simulink model "regulador_estabilidade"  (Simulink 7.9)
settings: Solver=ode4  SolverMode=SingleTasking  StartTime=0.0  StopTime=12  FixedStep=0.1  RelTol=1e-3
StartFcn:
  | clc
undefined symbols (not defined in the file or in its folder): A, Ac, Aeq, Aqp, B, Bc, Hn, Hqp, Phiu, Q, R, T
settings Model: Creator=Kawakami  LastModifiedBy=Kawakami
settings DataIOCC: SignalLoggingName=sigsOut
settings OptimizationCC: BooleanDataType=off
settings DebuggingCC: SaveWithParameterizedLinksMsg=none  SignalResolutionControl=TryResolveAllWithWarning  SolverPrmCheckMsg=none  MultiTaskDSMMsg=warning  MultiTaskCondExecSysMsg=none  FcnCallInpInsideContextMsg=Use local settings  StrictBusMsg=None
settings HardwareCC: TargetUnknown=on
settings RTWCC: IncludeERTFirstTime=on
settings GRTTargetCC: CombineOutputUpdateFcns=off  GRTInterface=on

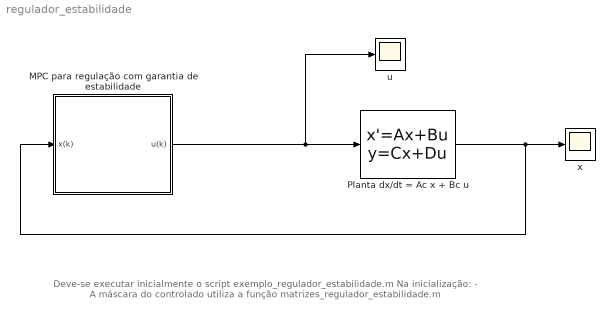
== system regulador_estabilidade ==
  note: Deve-se executar inicialmente o script exemplo_regulador_estabilidade.m
      |
      | Na inicialização:
      | - A máscara do controlado utiliza a função matrizes_regulador_estabilidade.m
  MPC para regulação com garantia de estabilidade : Subsystem  mask{Q=Q, R=R, N=10, A=A, B=B, ulim=[-0.2 0.2], xlim=[-2 2;-2 2], T=T}
      mask prompts: Q "Matriz de pesos dos estados Q (n x n)"; R "Matriz de pesos dos controle (R) (p x p)"; N "Horizonte de Predição (N)"; A "Matriz A (n x n)"; B "Matriz B (n x p)"; ulim "[umin, umax] (p x 2)"; xlim "[xmin, xmax] (n x 2)"; T "Periodo de amostragem"
      mask init:
      | [Phiu,Hn,Hqp,Aqp,Aeq] = matrizes_regulador_estabilidade(A,B,N,Q,R);
      | n = size(A,1);
      | p = size(B,2);
      | umin = ulim(:,1);
      | umax = ulim(:,2);
      | xmin = xlim(:,1);
      | xmax = xlim(:,2);
  "Planta dx/dt = Ac x + Bc u " : StateSpace  A=Ac  B=Bc  C=eye(size(A,1),size(A,1))  D=zeros(size(A,1),size(B,2))  X0=[1;0]
  u : Scope
      settings: TimeRange=12  YMin=-2  YMax=0.5  SaveName=y
  x : Scope
      settings: TimeRange=12  YMin=-1  YMax=2.5  SaveName=y6
  wires:
  MPC para regulação com garantia de estabilidade/1(u(k)) -> "Planta dx/dt = Ac x + Bc u "/1, u/1
  "Planta dx/dt = Ac x + Bc u "/1 -> MPC para regulação com garantia de estabilidade/1(x(k)), x/1

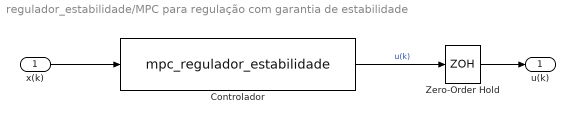
== system regulador_estabilidade/MPC para regulação com garantia de estabilidade ==
  x(k) : Inport
  Controlador : S-Function  FunctionName=mpc_regulador_estabilidade  Parameters=Phiu,Hn,Hqp,Aqp,Aeq,umax,umin,xmax,xmin,p,n,N,T  EnableBusSupport=off
  Zero-Order Hold : ZeroOrderHold  SampleTime=T
  u(k) : Outport
  wires:
  Zero-Order Hold/1 -> u(k)/1
  Controlador/1 -> Zero-Order Hold/1  "u(k)"
  x(k)/1 -> Controlador/1
